simulink model "GuiamentoOrbital"  (R2023b)
settings: Solver=FixedStepAuto  StartTime=0.0  StopTime=tf  FixedStep=step_modelo  RelTol=1e-8  AbsTol=abs_tol
settings Model: Creator=rodri  LastModifiedBy=rodri

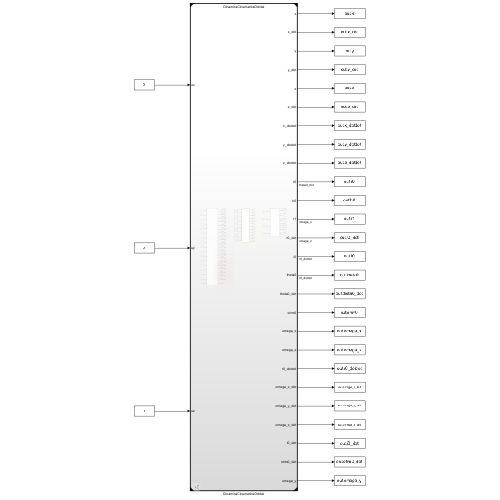
[thumbnail: Simulink's stored preview of the top-level diagram]
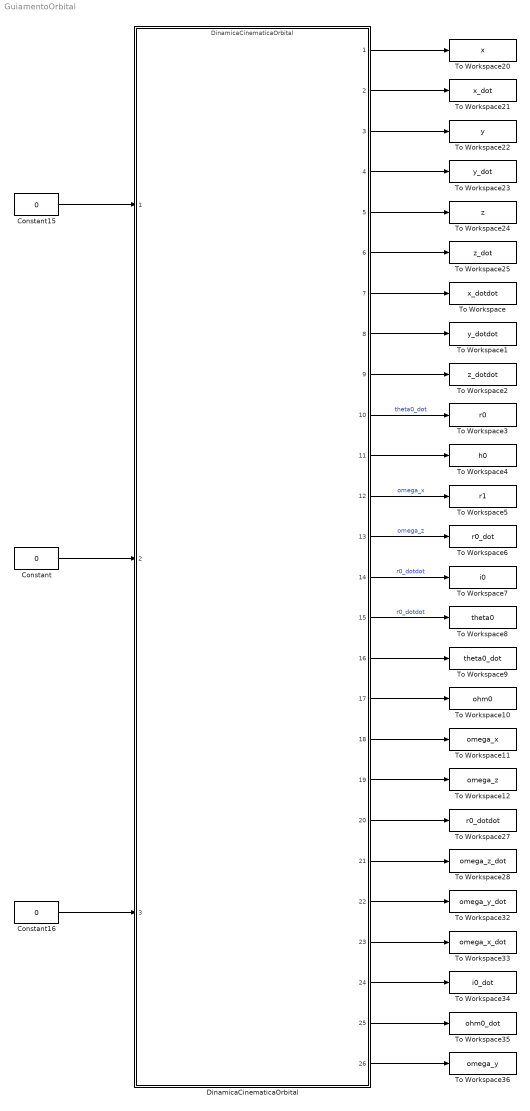
== system GuiamentoOrbital ==
  Constant : Constant  Value=0
  Constant15 : Constant  Value=0
  Constant16 : Constant  Value=0
  DinamicaCinematicaOrbital : ModelReference  ModelNameDialog=DinamicaCinematicaOrbital  ModelReferenceVersion=4.23
  To Workspace : ToWorkspace  VariableName=x_dotdot  SaveFormat=Timeseries  SampleTime=-1
  To Workspace1 : ToWorkspace  VariableName=y_dotdot  SaveFormat=Timeseries  SampleTime=-1
  To Workspace10 : ToWorkspace  VariableName=ohm0  SaveFormat=Timeseries  SampleTime=-1
  To Workspace11 : ToWorkspace  VariableName=omega_x  SaveFormat=Timeseries  SampleTime=-1
  To Workspace12 : ToWorkspace  VariableName=omega_z  SaveFormat=Timeseries  SampleTime=-1
  To Workspace2 : ToWorkspace  VariableName=z_dotdot  SaveFormat=Timeseries  SampleTime=-1
  To Workspace20 : ToWorkspace  VariableName=x  SaveFormat=Timeseries  SampleTime=-1
  To Workspace21 : ToWorkspace  VariableName=x_dot  SaveFormat=Timeseries  SampleTime=-1
  To Workspace22 : ToWorkspace  VariableName=y  SaveFormat=Timeseries  SampleTime=-1
  To Workspace23 : ToWorkspace  VariableName=y_dot  SaveFormat=Timeseries  SampleTime=-1
  To Workspace24 : ToWorkspace  VariableName=z  SaveFormat=Timeseries  SampleTime=-1
  To Workspace25 : ToWorkspace  VariableName=z_dot  SaveFormat=Timeseries  SampleTime=-1
  To Workspace27 : ToWorkspace  VariableName=r0_dotdot  SaveFormat=Timeseries  SampleTime=-1
  To Workspace28 : ToWorkspace  VariableName=omega_z_dot  SaveFormat=Timeseries  SampleTime=-1
  To Workspace3 : ToWorkspace  VariableName=r0  SaveFormat=Timeseries  SampleTime=-1
  To Workspace32 : ToWorkspace  VariableName=omega_y_dot  SaveFormat=Timeseries  SampleTime=-1
  To Workspace33 : ToWorkspace  VariableName=omega_x_dot  SaveFormat=Timeseries  SampleTime=-1
  To Workspace34 : ToWorkspace  VariableName=i0_dot  SaveFormat=Timeseries  SampleTime=-1
  To Workspace35 : ToWorkspace  VariableName=ohm0_dot  SaveFormat=Timeseries  SampleTime=-1
  To Workspace36 : ToWorkspace  VariableName=omega_y  SaveFormat=Timeseries  SampleTime=-1
  To Workspace4 : ToWorkspace  VariableName=h0  SaveFormat=Timeseries  SampleTime=-1
  To Workspace5 : ToWorkspace  VariableName=r1  SaveFormat=Timeseries  SampleTime=-1
  To Workspace6 : ToWorkspace  VariableName=r0_dot  SaveFormat=Timeseries  SampleTime=-1
  To Workspace7 : ToWorkspace  VariableName=i0  SaveFormat=Timeseries  SampleTime=-1
  To Workspace8 : ToWorkspace  VariableName=theta0  SaveFormat=Timeseries  SampleTime=-1
  To Workspace9 : ToWorkspace  VariableName=theta0_dot  SaveFormat=Timeseries  SampleTime=-1
  wires:
  Constant/1 -> DinamicaCinematicaOrbital/2
  Constant15/1 -> DinamicaCinematicaOrbital/1
  Constant16/1 -> DinamicaCinematicaOrbital/3
  DinamicaCinematicaOrbital/6 -> To Workspace25/1
  DinamicaCinematicaOrbital/1 -> To Workspace20/1
  DinamicaCinematicaOrbital/3 -> To Workspace22/1
  DinamicaCinematicaOrbital/5 -> To Workspace24/1
  DinamicaCinematicaOrbital/4 -> To Workspace23/1
  DinamicaCinematicaOrbital/2 -> To Workspace21/1
  DinamicaCinematicaOrbital/26 -> To Workspace36/1
  DinamicaCinematicaOrbital/25 -> To Workspace35/1
  DinamicaCinematicaOrbital/24 -> To Workspace34/1
  DinamicaCinematicaOrbital/23 -> To Workspace33/1
  DinamicaCinematicaOrbital/22 -> To Workspace32/1
  DinamicaCinematicaOrbital/21 -> To Workspace28/1
  DinamicaCinematicaOrbital/20 -> To Workspace27/1
  DinamicaCinematicaOrbital/19 -> To Workspace12/1
  DinamicaCinematicaOrbital/18 -> To Workspace11/1
  DinamicaCinematicaOrbital/17 -> To Workspace10/1
  DinamicaCinematicaOrbital/16 -> To Workspace9/1
  DinamicaCinematicaOrbital/15 -> To Workspace8/1  "r0_dotdot"
  DinamicaCinematicaOrbital/14 -> To Workspace7/1  "r0_dotdot"
  DinamicaCinematicaOrbital/13 -> To Workspace6/1  "omega_z"
  DinamicaCinematicaOrbital/12 -> To Workspace5/1  "omega_x"
  DinamicaCinematicaOrbital/11 -> To Workspace4/1
  DinamicaCinematicaOrbital/10 -> To Workspace3/1  "theta0_dot"
  DinamicaCinematicaOrbital/9 -> To Workspace2/1
  DinamicaCinematicaOrbital/8 -> To Workspace1/1
  DinamicaCinematicaOrbital/7 -> To Workspace/1
